simulink model "CurrentControl"  (R2019b)
settings: Solver=VariableStepAuto  StartTime=0.0  StopTime=0.5  MaxStep=0.5/25000  RelTol=1e-3
undefined symbols (not defined in the file): B, J, Lm, Rm
libraries: simulink x2
settings Model: Creator=Mark  LastModifiedBy=Mark

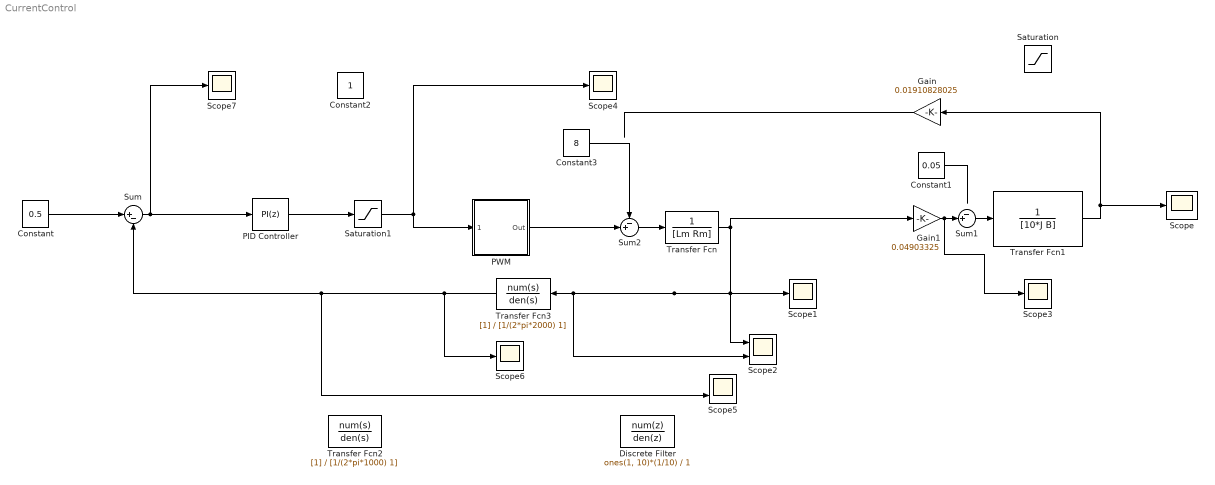
== system CurrentControl ==
  Constant : Constant  Value=0.5
  Constant1 : Constant  Value=0.05
  Constant2 : Constant
  Constant3 : Constant  Value=8
  Discrete Filter : DiscreteFilter  Numerator=ones(1, 10)*(1/10)  Denominator=1  SampleTime=1/100000
  Gain : Gain  Gain=0.01910828025
  Gain1 : Gain  Gain=0.04903325
  PID Controller : simulink/Continuous/PID Controller  Controller=PI  Form=Parallel  TimeDomain=Discrete-time  SampleTime=1/5000  IntegratorMethod=Forward Euler  FilterMethod=Forward Euler  ControllerParametersSource=internal  P=0.960142890292665  I=995.694725887012  D=0  UseFilter=on  N=100  TunerSelectOption=Transfer Function Based (PID Tuner App)  InitialConditionSource=internal  InitialConditionForIntegrator=0  InitialConditionForFilter=0  DifferentiatorICPrevScaledInput=0  ExternalReset=none  TrackingMode=off  Kt=1  LimitOutput=off  UpperSaturationLimit=inf  LowerSaturationLimit=-inf  LinearizeAsGain=on  AntiWindupMode=none  Kb=1  POutMin=[]  POutMax=[]  IOutMin=[]  IOutMax=[]  DOutMin=[]  DOutMax=[]  NOutMin=[]  NOutMax=[]  SumOutMin=[]  SumOutMax=[]  SaturationOutMin=[]  SaturationOutMax=[]  PParamMin=[]  PParamMax=[]  IParamMin=[]  IParamMax=[]  DParamMin=[]  DParamMax=[]  NParamMin=[]  NParamMax=[]  KbParamMin=[]  KbParamMax=[]  KtParamMin=[]  KtParamMax=[]  KbOutMin=[]  KbOutMax=[]  KtOutMin=[]  KtOutMax=[]  IntegratorOutMin=[]  IntegratorOutMax=[]  FilterOutMin=[]  FilterOutMax=[]  SumI1OutMin=[]  SumI1OutMax=[]  SumI2OutMin=[]  SumI2OutMax=[]  SumI3OutMin=[]  SumI3OutMax=[]  SumI4OutMin=[]  SumI4OutMax=[]  SumDOutMin=[]  SumDOutMax=[]  DifferentiatorOutMin=[]  DifferentiatorOutMax=[]  FilterDiffOutCoefMin=[]  FilterDiffOutCoefMax=[]  ReciprocalOutMin=[]  ReciprocalOutMax=[]  SumDenOutMin=[]  SumDenOutMax=[]  SumNumOutMin=[]  SumNumOutMax=[]  DivideOutMin=[]  DivideOutMax=[]  IntegratorContinuousStateAttributes=''  IntegratorStateMustResolveToSignalObject=off  IntegratorRTWStateStorageClass=Auto  FilterContinuousStateAttributes=''  FilterStateMustResolveToSignalObject=off  FilterRTWStateStorageClass=Auto  ParallelPVariant=InternalParameters  IdealPVariant=Disabled  IVariant=InternalParameters  DVariant=Disabled  IntegratorVariant=Discrete  SatVariant=Disabled  AWVariant=Passthrough  PCopyVariant=Disabled  TRVariant=Disabled  FdbkBlocksVariant=Forward  IdealPFdbkVariant=Disabled  SatFdbkVariant=Disabled  DerivativeFilterVariant=Disabled  NVariant=Disabled  NCopyVariant=Disabled_SignalSpec  FilterICVariant=Disabled  IntegratorICVariant=InternalICs  ExternalResetVariant=Disabled  TRSumVariant=Passthrough  SumFdbkVariant=Disabled  SumVariant=Sum_PI
  PWM : Subsystem
  Saturation : Saturate  UpperLimit=628  LowerLimit=-628
  Saturation1 : Saturate  UpperLimit=12  LowerLimit=-12
  Scope{,1,3..4,6..7} (6 alike) : Scope
  Scope2 : Scope  NumInputPorts=2
  Scope5 : Scope  NumInputPorts=2
  Sum : Sum  Inputs=|+-
  Sum1 : Sum  Inputs=-+|
  Sum2 : Sum  Inputs=-+|
  Transfer Fcn : TransferFcn  Denominator=[Lm Rm]
  Transfer Fcn1 : TransferFcn  Denominator=[10*J B]
  Transfer Fcn2 : TransferFcn  Denominator=[1/(2*pi*1000) 1]
  Transfer Fcn3 : TransferFcn  Denominator=[1/(2*pi*2000) 1]
  wires:
  Gain1/1 -> Scope3/1, Sum1/2
  Sum1/1 -> Transfer Fcn1/1
  Constant1/1 -> ?
  Gain/1 -> ?
  Transfer Fcn1/1 -> Gain/1, Scope/1
  Sum2/1 -> Transfer Fcn/1
  Sum/1 -> PID Controller/1, Scope7/1
  Constant/1 -> Sum/1
  PID Controller/1 -> Saturation1/1
  Transfer Fcn/1 -> Gain1/1, Transfer Fcn3/1, Scope2/2, Scope1/1, Scope2/1
  Transfer Fcn3/1 -> Scope5/2, Sum/2, Scope6/1
  Saturation1/1 -> Scope4/1, PWM/1(Voltage)
  PWM/1(Out) -> Sum2/2
  Constant3/1 -> Sum2/1

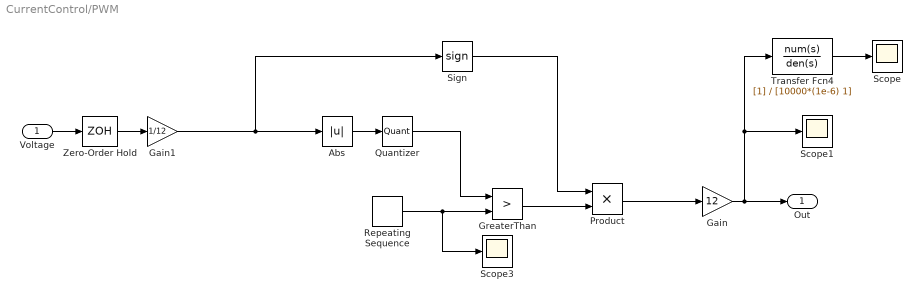
== system CurrentControl/PWM ==
  Voltage : Inport
  Abs : Abs
  Gain : Gain  Gain=12
  Gain1 : Gain  Gain=1/12
  GreaterThan : RelationalOperator  Operator=>  OutDataTypeStr=boolean  RndMeth=Simplest
  Product : Product
  Quantizer : Quantizer  QuantizationInterval=1/4096
  Repeating Sequence : simulink/Sources/Repeating Sequence  rep_seq_t=[0 1/25000]  rep_seq_y=[0 1]
  Scope : Scope
  Scope1 : Scope
  Scope3 : Scope
  Sign : Signum
  Transfer Fcn4 : TransferFcn  Denominator=[10000*(1e-6) 1]
  Zero-Order Hold : ZeroOrderHold  SampleTime=1/10000
  Out : Outport
  wires:
  Repeating Sequence/1 -> Scope3/1, GreaterThan/2
  Voltage/1 -> Zero-Order Hold/1
  GreaterThan/1 -> Product/2
  Abs/1 -> Quantizer/1
  Sign/1 -> Product/1
  Product/1 -> Gain/1
  Gain/1 -> Transfer Fcn4/1, Scope1/1, Out/1
  Gain1/1 -> Sign/1, Abs/1
  Zero-Order Hold/1 -> Gain1/1
  Transfer Fcn4/1 -> Scope/1
  Quantizer/1 -> GreaterThan/1
